simulink model "drone_PID_PWM"  (Simulink 10.0)
settings: Solver=ode45  StartTime=0.0  StopTime=100  FixedStep=1e-3  RelTol=1e-5  EnableMultiTasking=on
values from neighbouring files (symbols this model uses):
  A = [0 0 1 0;0 0 0 1;0 0 -Kax/M 0;0 0 0 -Kay/M]    [modello_drone.m]
  B = [0 0;0 0;1/M 0;0 1/M]    [modello_drone.m]
  C = [1 0 0 0;0 1 0 0]    [modello_drone.m]
  D = zeros(2,5)    [modello_drone.m]
  G = [0 0 0 -1]'    [modello_drone.m]
  Mmax = 2,Mn=1.8    [modello_drone.m]
undefined symbols (not defined in the file or in its folder): Mn
libraries: simulink x3, simulink_need_slupdate x1
settings Model: Creator=prof. G. Celentano  LastModifiedBy=giuseppericcio
settings DataIOCC: LimitDataPoints=on  SignalLoggingSaveFormat=ModelDataLogs  SignalLoggingName=sigsOut
settings OptimizationCC: ExpressionDepthLimit=2147483647  InitFltsAndDblsToZero=on
settings DebuggingCC: SaveWithParameterizedLinksMsg=none  SignalResolutionControl=TryResolveAllWithWarning  MultiTaskDSMMsg=warning  MultiTaskCondExecSysMsg=none  FcnCallInpInsideContextMsg=warning  StateNameClashWarn=warning
settings HardwareCC: TargetUnknown=on
settings GRTTargetCC: TargetFcnLib=ansi_tfl_tmw.mat

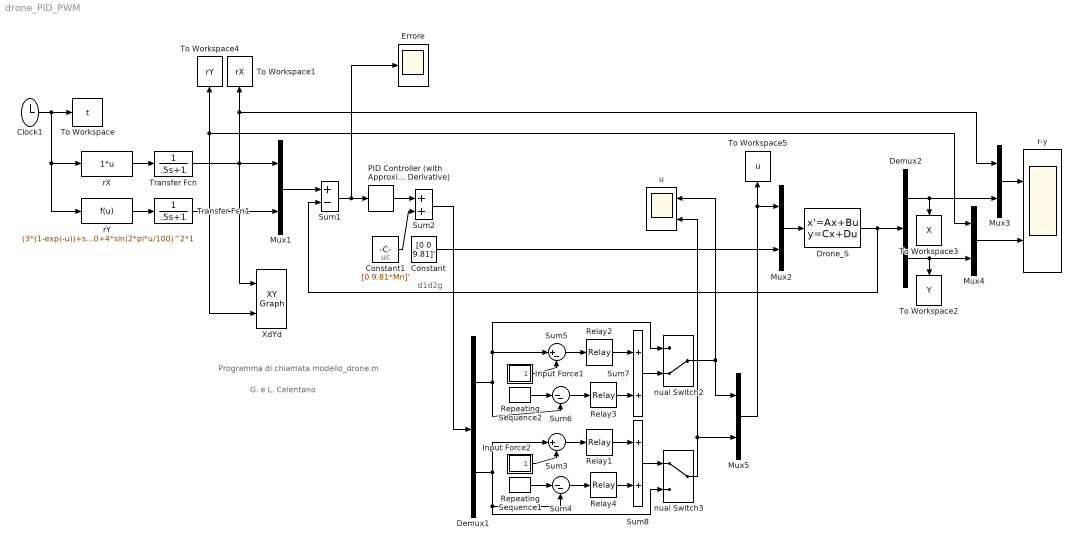
== system drone_PID_PWM ==
  note: G. e L. Celentano
  note: Programma di chiamata modello_drone.m
  note: d1d2g
  note: uc
  " Errore" : Scope
  " XdYd " : simulink/Sinks/XY Graph  xmin=0  xmax=100  ymin=0  ymax=5  st=-1
  Clock1 : Clock
  Constant : Constant  Value=[0 0 9.81]'
  Constant1 : Constant  Value=[0 9.81*Mn]'
  Demux1 : Demux  Outputs=2
  Demux2 : Demux  Outputs=2
  Drone_S : StateSpace  A=A  B=[B E G]  C=C  D=D  InitialCondition=0
  Input Force1 : Subsystem  mask(Repeating table){rep_seq_t=[0  .01], rep_seq_y=[0 10 ]}
      mask prompts: rep_seq_t "Time values:"; rep_seq_y "Output values:"
      mask help: Repeating table.
      mask init:
      | period = max(rep_seq_t);
      mask Help: Repeats cycle given in table. Time values should be monotonically increasing.
      mask Display: plot([rep_seq_t,rep_seq_t+period,rep_seq_t+2*period,rep_seq_t(1)+3*period],[rep_seq_y,rep_seq_y,rep_seq_y,rep_seq_y(1)])
  Input Force2 : Subsystem  mask(Repeating table){rep_seq_t=[0  .01], rep_seq_y=[0 40 ]}
      mask prompts: rep_seq_t "Time values:"; rep_seq_y "Output values:"
      mask help: Repeating table.
      mask init:
      | period = max(rep_seq_t);
      mask Help: Repeats cycle given in table. Time values should be monotonically increasing.
      mask Display: plot([rep_seq_t,rep_seq_t+period,rep_seq_t+2*period,rep_seq_t(1)+3*period],[rep_seq_y,rep_seq_y,rep_seq_y,rep_seq_y(1)])
  Mux{1,3..5} (4 alike) : Mux  Inputs=[1 1]
  Mux2 : Mux  Inputs=[2 3]
  PID Controller (with Approximate Derivative) : simulink_need_slupdate/PID Controller (with Approximate Derivative)  P=Mmax*6*10^2  I=Mmax*4*10^3  D=Mmax*3*10  N=100
      settings: SourceProductName=Simulink  SourceProductBaseCode=SL
  Relay1 : Relay  OnSwitchValue=0  OffSwitchValue=0  OnOutputValue=40
  Relay2 : Relay  OnSwitchValue=0  OffSwitchValue=0  OnOutputValue=10
  Relay3 : Relay  OnSwitchValue=0  OffSwitchValue=0  OnOutputValue=-10
  Relay4 : Relay  OnSwitchValue=0  OffSwitchValue=0  OnOutputValue=-40
  Repeating Sequence1 : simulink/Sources/Repeating Sequence  rep_seq_t="[0  .01]"  rep_seq_y=[0 40]
  Repeating Sequence2 : simulink/Sources/Repeating Sequence  rep_seq_t="[0  .01]"  rep_seq_y=[0 10]
  Sum1 : Sum  Inputs=+-  SaturateOnIntegerOverflow=on  InputSameDT=on  OutDataTypeStr=Inherit: Same as first input
  Sum2 : Sum  SaturateOnIntegerOverflow=on  InputSameDT=on  OutDataTypeStr=Inherit: Same as first input
  Sum3 : Sum  Inputs=|+-  SaturateOnIntegerOverflow=on
  Sum4 : Sum  Inputs=|--  SaturateOnIntegerOverflow=on
  Sum5 : Sum  Inputs=|+-  SaturateOnIntegerOverflow=on
  Sum6 : Sum  Inputs=|--  SaturateOnIntegerOverflow=on
  Sum7 : Sum  SaturateOnIntegerOverflow=on
  Sum8 : Sum  SaturateOnIntegerOverflow=on
  To Workspace : ToWorkspace  VariableName=t  SampleTime=-1
  To Workspace1 : ToWorkspace  VariableName=rX  SampleTime=-1
  To Workspace2 : ToWorkspace  VariableName=Y  SampleTime=-1
  To Workspace3 : ToWorkspace  VariableName=X  SampleTime=-1
  To Workspace4 : ToWorkspace  VariableName=rY  SampleTime=-1
  To Workspace5 : ToWorkspace  VariableName=u  SampleTime=-1
  Transfer Fcn : TransferFcn  Denominator=[.5 1]
  Transfer Fcn1 : TransferFcn  Denominator=[.5 1]
  nual Switch2 : ManualSwitch  CurrentSetting=0
  nual Switch3 : ManualSwitch
  r-y : Scope  NumInputPorts=2
  rX : Fcn  Expr=1*u
  rY : Fcn  Expr=(3*(1-exp(-u))+sin(2*pi/20*u))*0+4*sin(2*pi*u/100)^2*1
  u : Scope  NumInputPorts=2
  wires:
  Drone_S/1 -> Demux2/1, Sum1/2
  Mux2/1 -> Drone_S/1
  Mux3/1 -> r-y/1
  Mux4/1 -> r-y/2
  Demux2/1 -> Mux3/2, To Workspace3/1
  Demux2/2 -> Mux4/2, To Workspace2/1
  Clock1/1 -> To Workspace/1, rX/1, rY/1
  Transfer Fcn/1 -> " XdYd "/1, To Workspace1/1, Mux3/1, Mux1/1
  rX/1 -> Transfer Fcn/1
  rY/1 -> Transfer Fcn1/1
  Transfer Fcn1/1 -> " XdYd "/2, To Workspace4/1, Mux4/1, Mux1/2
  Constant/1 -> Mux2/2
  Mux1/1 -> Sum1/1
  Sum1/1 -> " Errore"/1, PID Controller (with Approximate Derivative)/1
  PID Controller (with Approximate Derivative)/1 -> Sum2/1
  Constant1/1 -> Sum2/2
  Sum2/1 -> Demux1/1
  Input Force1/1(out_1) -> Sum5/2
  Demux1/1 -> Sum6/2, Sum5/1, nual Switch2/1
  Sum5/1 -> Relay2/1
  Repeating Sequence2/1 -> Sum6/1
  Sum6/1 -> Relay3/1
  Relay2/1 -> Sum7/1
  Relay3/1 -> Sum7/2
  Input Force2/1(out_1) -> Sum3/2
  Demux1/2 -> Sum3/1, Sum4/2, nual Switch3/2
  Sum3/1 -> Relay1/1
  Repeating Sequence1/1 -> Sum4/1
  Sum4/1 -> Relay4/1
  Relay1/1 -> Sum8/1
  Relay4/1 -> Sum8/2
  Mux5/1 -> Mux2/1, To Workspace5/1
  Sum7/1 -> nual Switch2/2
  Sum8/1 -> nual Switch3/1
  nual Switch2/1 -> Mux5/1, u/1
  nual Switch3/1 -> Mux5/2, u/2

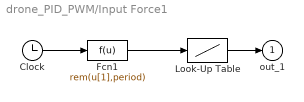
== system drone_PID_PWM/Input Force1 ==
  Clock : Clock
  Fcn1 : Fcn  Expr=rem(u[1],period)
  Look-Up Table : Lookup  InputValues=rep_seq_t  Table=rep_seq_y  SaturateOnIntegerOverflow=on
  out_1 : Outport  InitialOutput=0
  wires:
  Fcn1/1 -> Look-Up Table/1
  Clock/1 -> Fcn1/1
  Look-Up Table/1 -> out_1/1

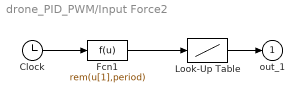
== system drone_PID_PWM/Input Force2 ==
  Clock : Clock
  Fcn1 : Fcn  Expr=rem(u[1],period)
  Look-Up Table : Lookup  InputValues=rep_seq_t  Table=rep_seq_y  SaturateOnIntegerOverflow=on
  out_1 : Outport  InitialOutput=0
  wires:
  Fcn1/1 -> Look-Up Table/1
  Clock/1 -> Fcn1/1
  Look-Up Table/1 -> out_1/1
